simulink model "test"  (R2022a)
settings: Solver=FixedStepDiscrete  StartTime=0.0  StopTime=inf  RelTol=1e-3  EnableMultiTasking=on
InitFcn:
  | run('busObjects.m')
model workspace (MAT data in the model file):
  omega = 8
  zeta = 0.05
libraries: aru_toolbox x1
settings Model: SimulationMode=external  Creator=Mechatronics  LastModifiedBy=Mechatronics
settings SolverCC: ConcurrentTasks=on  AlgebraicLoopSolver=TrustRegion  PositivePriorityOrder=on  InsertRTBMode=Never (minimum delay)
settings DataIOCC: SaveFormat=Array  SaveState=on  SignalLoggingName=logsOut
settings OptimizationCC: BlockReduction=off  BooleanDataType=off  OptimizeBlockIOStorage=off  BufferReuse=off  GlobalBufferReuse=off  ExpressionFolding=off  LocalBlockOutputs=off  InitFltsAndDblsToZero=on  OptimizeDataStoreBuffers=off  BusAssignmentInplaceUpdate=off
settings DebuggingCC: SaveWithParameterizedLinksMsg=none  UnderspecifiedInitializationDetection=Classic  MergeDetectMultiDrivingBlocksExec=none  CheckExecutionContextPreStartOutputMsg=on  SignalResolutionControl=TryResolveAllWithWarning  TasksWithSamePriorityMsg=none  UnconnectedInputMsg=warning  UnconnectedOutputMsg=warning  UnconnectedLineMsg=warning  SFUnexpectedBacktrackingDiag=warning  SFNoUnconditionalDefaultTransitionDiag=warning  SFExecutionAtInitializationDiag=none  SFMachineParentedDataDiag=warning  ArithmeticOperatorsInVariantConditions=warning
settings HardwareCC: ProdBitPerLong=64  ProdLongLongMode=on  ProdHWDeviceType=Intel->x86-64 (Linux 64)
settings ModelReferenceCC: PropagateSignalLabelsOutOfModel=off
settings SFSimCC: SimUseLocalCustomCode=off  SimTargetLang=C++
settings RTWCC: Description=Simulink Real-Time  SystemTargetFile=slrealtime.tlc  TemplateMakefile=slrealtime_default_tmf  RTWUseLocalCustomCode=off  Toolchain=Simulink Real-Time Toolchain  BuildConfiguration=Faster Runs  CodeExecutionProfiling=on  TargetLang=C++  DLArmComputeVersion=19.05
settings CodeAppCC: StateflowObjectComments=on
settings SimulinkRealTimeTargetCC: MATLABClassNameForMDSCustomization=Simulink.SoftwareTarget.GRTCustomization  UseGCCFastMath=on
settings ConfigComp: CovMetricSettings=dw  CovSaveCumulativeToWorkspaceVar=on  CovSaveSingleToWorkspaceVar=on  CovExternalEMLEnable=off  CovSFcnEnable=off

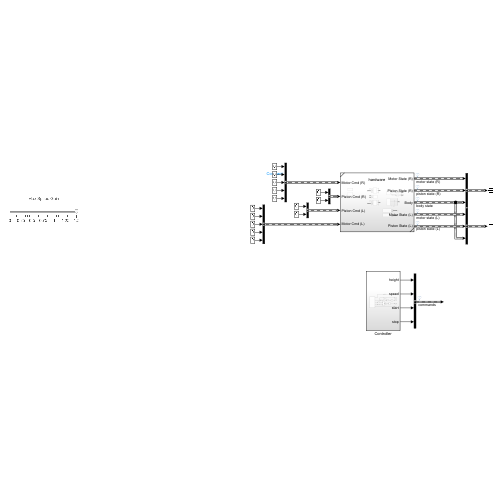
[thumbnail: Simulink's stored preview of the top-level diagram]
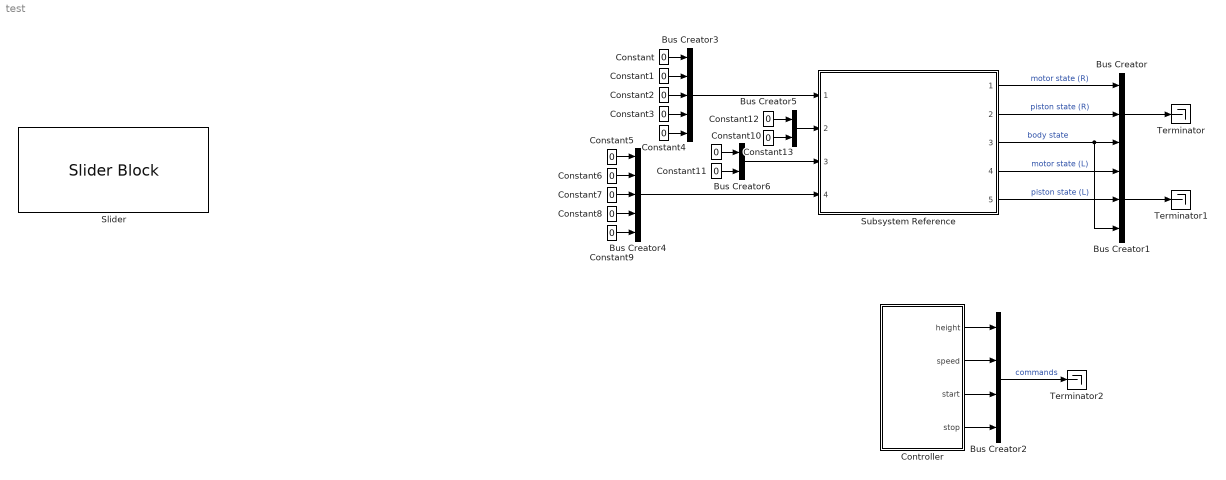
== system test ==
  Bus Creator : BusCreator  Inputs=3  OutDataTypeStr=Bus: State  NonVirtualBus=on
      settings: InheritFromInputs=off
  Bus Creator1 : BusCreator  Inputs=3  OutDataTypeStr=Bus: State  NonVirtualBus=on
      settings: InheritFromInputs=off
  Bus Creator2 : BusCreator  Inputs=4  OutDataTypeStr=Bus: Command  NonVirtualBus=on
      settings: InheritFromInputs=off
  Bus Creator3 : BusCreator  Inputs=5  OutDataTypeStr=Bus: MotorCmd  NonVirtualBus=on
      settings: InheritFromInputs=off
  Bus Creator4 : BusCreator  Inputs=5  OutDataTypeStr=Bus: MotorCmd  NonVirtualBus=on
      settings: InheritFromInputs=off
  Bus Creator5 : BusCreator  Inputs=2  OutDataTypeStr=Bus: PistonCmd  NonVirtualBus=on
      settings: InheritFromInputs=off
  Bus Creator6 : BusCreator  Inputs=2  OutDataTypeStr=Bus: PistonCmd  NonVirtualBus=on
      settings: InheritFromInputs=off
  Constant{,1..13} (14 alike) : Constant  Value=0
  Controller : Subsystem
  Slider : SliderBlock  ScaleMax=1.5
  Subsystem Reference : Subsystem  ReferencedSubsystem=hardware
  Terminator : Terminator
  Terminator1 : Terminator
  Terminator2 : Terminator
  wires:
  Subsystem Reference/4 -> Bus Creator1/1  "motor state (L)"
  Subsystem Reference/5 -> Bus Creator1/2  "piston state (L)"
  Subsystem Reference/3 -> Bus Creator1/3, Bus Creator/3  "body state"
  Subsystem Reference/2 -> Bus Creator/2  "piston state (R)"
  Subsystem Reference/1 -> Bus Creator/1  "motor state (R)"
  Bus Creator2/1 -> Terminator2/1  "commands"
  Controller/2(speed) -> Bus Creator2/2
  Controller/1(height) -> Bus Creator2/1
  Controller/3(start) -> Bus Creator2/3
  Controller/4(stop) -> Bus Creator2/4
  Bus Creator/1 -> Terminator/1
  Bus Creator1/1 -> Terminator1/1
  Bus Creator3/1 -> Subsystem Reference/1
  Constant/1 -> Bus Creator3/1
  Constant1/1 -> Bus Creator3/2
  Constant2/1 -> Bus Creator3/3
  Constant3/1 -> Bus Creator3/4
  Constant4/1 -> Bus Creator3/5
  Constant6/1 -> Bus Creator4/2
  Constant8/1 -> Bus Creator4/4
  Constant7/1 -> Bus Creator4/3
  Bus Creator4/1 -> Subsystem Reference/4
  Constant5/1 -> Bus Creator4/1
  Constant9/1 -> Bus Creator4/5
  Bus Creator5/1 -> Subsystem Reference/2
  Bus Creator6/1 -> Subsystem Reference/3
  Constant10/1 -> Bus Creator6/1
  Constant11/1 -> Bus Creator6/2
  Constant12/1 -> Bus Creator5/1
  Constant13/1 -> Bus Creator5/2

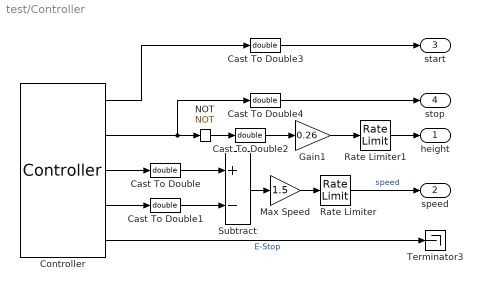
== system test/Controller ==
  Cast To Double{,1..4} (5 alike) : DataTypeConversion  OutDataTypeStr=double  SaturateOnIntegerOverflow=off  RndMeth=Floor
  Controller : aru_toolbox/Controller
      link override "LVTTL digital input ": parInternalModuleId=1
      settings: SourceProductName=ARU Toolbox
  Gain1 : Gain  Gain=0.26
  Max Speed : Gain  Gain=1.5
  NOT : Logic  Operator=NOT  IconShape=distinctive  AllPortsSameDT=off  OutDataTypeStr=boolean
  Rate Limiter : RateLimiter  RisingSlewLimit=0.5  FallingSlewLimit=-0.5  SampleTimeMode=inherited
  Rate Limiter1 : RateLimiter  RisingSlewLimit=0.05  FallingSlewLimit=-0.05  SampleTimeMode=inherited  InitialCondition=0.26
  Subtract : Sum  Inputs=+-
  Terminator3 : Terminator
  height : Outport
  speed : Outport  Port=2
  start : Outport  Port=3
  stop : Outport  Port=4
  wires:
  Gain1/1 -> Rate Limiter1/1
  Rate Limiter/1 -> speed/1  "speed"
  Subtract/1 -> Max Speed/1
  Controller/5 -> Terminator3/1  "E-Stop"
  Controller/2 -> Cast To Double4/1, NOT/1
  Controller/3 -> Cast To Double/1
  Max Speed/1 -> Rate Limiter/1
  Controller/4 -> Cast To Double1/1
  Cast To Double/1 -> Subtract/1
  Cast To Double1/1 -> Subtract/2
  Controller/1 -> Cast To Double3/1
  Rate Limiter1/1 -> height/1
  Cast To Double3/1 -> start/1
  NOT/1 -> Cast To Double2/1
  Cast To Double2/1 -> Gain1/1
  Cast To Double4/1 -> stop/1
